simulink model "SCG007C_TC_Development_r01"  (R2017b)
settings: Solver=VariableStepAuto  StartTime=0.0  StopTime=10.0  RelTol=1e-3
values from neighbouring files (symbols this model uses):
  MP_SLIP_val = [ ... (first row only)    [Calibration_r01_v01.m]
  MP_SLIP_x1 = [0.000 0.500 0.750 1.000 1.250 1.500 1.750 2.000 2.500]./2.5.*100    [Calibration_r01_v01.m]
  MP_SLIP_x2 = [0	1	2	3	4	5	6	7	8	9	10	11	12]    [Calibration_r01_v01.m]
  MP_SLIPIP_DSLIP_val = [ ... (first row only)    [Calibration_r01_v01.m]
  MP_SLIPIP_DSLIP_x1 = [0.0 20.0 40.0 60.0 70.0 80.0 90.0 100.0 110.0 120.0 140.0]    [Calibration_r01_v01.m]
  MP_SLIPIP_DSLIP_x2 = [-4.0 -2.0 -1.0 -0.6 0.0 0.1 0.5 3.0 5.0]    [Calibration_r01_v01.m]
  MP_SLIPPP_DSLIP_val = [ ... (first row only)    [Calibration_r01_v01.m]
  MP_SLIPPP_DSLIP_x1 = [0.0 20.0 40.0 60.0 70.0 80.0 90.0 100.0 110.0 120.0 140.0]    [Calibration_r01_v01.m]
  MP_SLIPPP_DSLIP_x2 = [-4.0 -2.0 -1.0 -0.6 0.0 0.1 0.5 3.0 5.0]    [Calibration_r01_v01.m]
undefined symbols (not defined in the file or in its folder): Engine, Standard_Input_Bus, TCS, vicrt_initcallback, vicrt_initmexcallback, vicrt_simulationmanager
libraries: simulink x7, simulink_extras x1
(part 2 of 5)

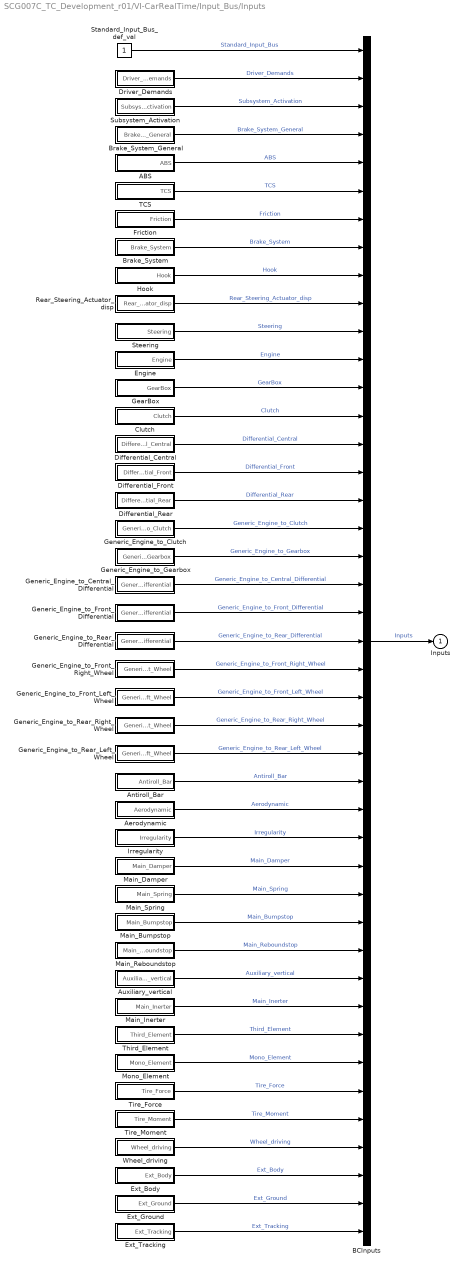
== system SCG007C_TC_Development_r01/VI-CarRealTime/Input_Bus/Inputs ==
  ABS : Subsystem
  Aerodynamic : Subsystem
  Antiroll_Bar : Subsystem
  Auxiliary_vertical : Subsystem
  BCInputs : BusCreator  Inputs=43
  Brake_System : Subsystem
  Brake_System_General : Subsystem
  Clutch : Subsystem
  Differential_Central : Subsystem
  Differential_Front : Subsystem
  Differential_Rear : Subsystem
  Driver_Demands : Subsystem
  Engine : Subsystem
  Ext_Body : Subsystem
  Ext_Ground : Subsystem
  Ext_Tracking : Subsystem
  Friction : Subsystem
  GearBox : Subsystem
  Generic_Engine_to_Central_Differential : Subsystem
  Generic_Engine_to_Clutch : Subsystem
  Generic_Engine_to_Front_Differential : Subsystem
  Generic_Engine_to_Front_Left_Wheel : Subsystem
  Generic_Engine_to_Front_Right_Wheel : Subsystem
  Generic_Engine_to_Gearbox : Subsystem
  Generic_Engine_to_Rear_Differential : Subsystem
  Generic_Engine_to_Rear_Left_Wheel : Subsystem
  Generic_Engine_to_Rear_Right_Wheel : Subsystem
  Hook : Subsystem
  Irregularity : Subsystem
  Main_Bumpstop : Subsystem
  Main_Damper : Subsystem
  Main_Inerter : Subsystem
  Main_Reboundstop : Subsystem
  Main_Spring : Subsystem
  Mono_Element : Subsystem
  Rear_Steering_Actuator_disp : Subsystem
  Standard_Input_Bus_def_val : Constant
  Steering : Subsystem
  Subsystem_Activation : Subsystem
  TCS : Subsystem
  Third_Element : Subsystem
  Tire_Force : Subsystem
  Tire_Moment : Subsystem
  Wheel_driving : Subsystem
  Inputs : Outport
  wires:
  BCInputs/1 -> Inputs/1  "Inputs"
  Standard_Input_Bus_def_val/1 -> BCInputs/1  "Standard_Input_Bus"
  Driver_Demands/1(Driver_Demands) -> BCInputs/2  "Driver_Demands"
  Subsystem_Activation/1(Subsystem_Activation) -> BCInputs/3  "Subsystem_Activation"
  Brake_System_General/1(Brake_System_General) -> BCInputs/4  "Brake_System_General"
  ABS/1(ABS) -> BCInputs/5  "ABS"
  TCS/1(TCS) -> BCInputs/6  "TCS"
  Friction/1(Friction) -> BCInputs/7  "Friction"
  Brake_System/1(Brake_System) -> BCInputs/8  "Brake_System"
  Hook/1(Hook) -> BCInputs/9  "Hook"
  Rear_Steering_Actuator_disp/1(Rear_Steering_Actuator_disp) -> BCInputs/10  "Rear_Steering_Actuator_disp"
  Steering/1(Steering) -> BCInputs/11  "Steering"
  Engine/1(Engine) -> BCInputs/12  "Engine"
  GearBox/1(GearBox) -> BCInputs/13  "GearBox"
  Clutch/1(Clutch) -> BCInputs/14  "Clutch"
  Differential_Central/1(Differential_Central) -> BCInputs/15  "Differential_Central"
  Differential_Front/1(Differential_Front) -> BCInputs/16  "Differential_Front"
  Differential_Rear/1(Differential_Rear) -> BCInputs/17  "Differential_Rear"
  Generic_Engine_to_Clutch/1(Generic_Engine_to_Clutch) -> BCInputs/18  "Generic_Engine_to_Clutch"
  Generic_Engine_to_Gearbox/1(Generic_Engine_to_Gearbox) -> BCInputs/19  "Generic_Engine_to_Gearbox"
  Generic_Engine_to_Central_Differential/1(Generic_Engine_to_Central_Differential) -> BCInputs/20  "Generic_Engine_to_Central_Differential"
  Generic_Engine_to_Front_Differential/1(Generic_Engine_to_Front_Differential) -> BCInputs/21  "Generic_Engine_to_Front_Differential"
  Generic_Engine_to_Rear_Differential/1(Generic_Engine_to_Rear_Differential) -> BCInputs/22  "Generic_Engine_to_Rear_Differential"
  Generic_Engine_to_Front_Right_Wheel/1(Generic_Engine_to_Front_Right_Wheel) -> BCInputs/23  "Generic_Engine_to_Front_Right_Wheel"
  Generic_Engine_to_Front_Left_Wheel/1(Generic_Engine_to_Front_Left_Wheel) -> BCInputs/24  "Generic_Engine_to_Front_Left_Wheel"
  Generic_Engine_to_Rear_Right_Wheel/1(Generic_Engine_to_Rear_Right_Wheel) -> BCInputs/25  "Generic_Engine_to_Rear_Right_Wheel"
  Generic_Engine_to_Rear_Left_Wheel/1(Generic_Engine_to_Rear_Left_Wheel) -> BCInputs/26  "Generic_Engine_to_Rear_Left_Wheel"
  Antiroll_Bar/1(Antiroll_Bar) -> BCInputs/27  "Antiroll_Bar"
  Aerodynamic/1(Aerodynamic) -> BCInputs/28  "Aerodynamic"
  Irregularity/1(Irregularity) -> BCInputs/29  "Irregularity"
  Main_Damper/1(Main_Damper) -> BCInputs/30  "Main_Damper"
  Main_Spring/1(Main_Spring) -> BCInputs/31  "Main_Spring"
  Main_Bumpstop/1(Main_Bumpstop) -> BCInputs/32  "Main_Bumpstop"
  Main_Reboundstop/1(Main_Reboundstop) -> BCInputs/33  "Main_Reboundstop"
  Auxiliary_vertical/1(Auxiliary_vertical) -> BCInputs/34  "Auxiliary_vertical"
  Main_Inerter/1(Main_Inerter) -> BCInputs/35  "Main_Inerter"
  Third_Element/1(Third_Element) -> BCInputs/36  "Third_Element"
  Mono_Element/1(Mono_Element) -> BCInputs/37  "Mono_Element"
  Tire_Force/1(Tire_Force) -> BCInputs/38  "Tire_Force"
  Tire_Moment/1(Tire_Moment) -> BCInputs/39  "Tire_Moment"
  Wheel_driving/1(Wheel_driving) -> BCInputs/40  "Wheel_driving"
  Ext_Body/1(Ext_Body) -> BCInputs/41  "Ext_Body"
  Ext_Ground/1(Ext_Ground) -> BCInputs/42  "Ext_Ground"
  Ext_Tracking/1(Ext_Tracking) -> BCInputs/43  "Ext_Tracking"
